simulink model "UnusedModels"  (R2015a)
settings: Solver=ode45  StartTime=0.0  StopTime=10.0  RelTol=1e-3
values from neighbouring files (symbols this model uses):
  car_params = Simulink_Car_params    [TV2016_parameters.m]
  energyLimitControl = Simulink_energyLimit    [TV2016_parameters.m]
  settings = Simulink_Settings    [TV2016_parameters.m]
  speedEstimation = Simulink_speedEst    [TV2016_parameters.m]
  tractionControl = Simulink_tc    [TV2016_parameters.m]
  yawRateControl = Simulink_yawRate    [TV2016_parameters.m]
undefined symbols (not defined in the file or in its folder): canChannel, Use_Estimated_velocity
libraries: canlib x44, CarMaker4SL x33, canmsglib x28, simulink x6
(part 2 of 4)

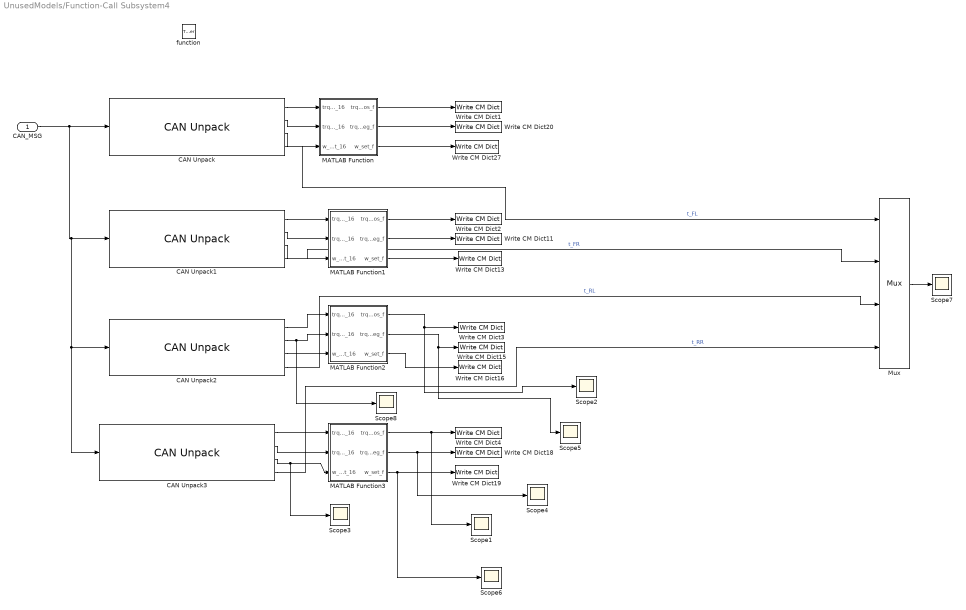
== system UnusedModels/Function-Call Subsystem4 ==
  CAN_MSG : Inport
  function : TriggerPort  TriggerType=function-call
  CAN Unpack : canmsglib/CAN Unpack  MsgList=(none)  MsgName=INV_FL  MsgIDType=Standard (11-bit identifier)  MsgIdentifier=CAN_ID_INV_FL  MsgLength=6  SignalInfo=trq_pos$0$16$1$1$1$0$1$0$-Inf$Inf$#trq_neg$16$16$1$1$1$0$1$0$-Inf$Inf$#w_set$32$16$1$1$1$0$1$0$-Inf$Inf$#  NSignals=3  IDPort=off  TimestampPort=on  ErrorPort=off  RemotePort=off  LengthPort=off  StatusPort=off  StartBits=str2num('[int32(0);int32(16);int32(32)]')  SignalSizes=str2num('[int32(16);int32(16);int32(16)]')  ByteOrders=str2num('[int32(1);int32(1);int32(1)]')  DataTypes=str2num('[int32(1);int32(1);int32(1)]')  MultiplexTypes=str2num('[int32(1);int32(1);int32(1)]')  MultiplexValues=str2num('[double(0);double(0);double(0)]')  Factors=str2num('[double(1);double(1);double(1)]')  Offsets=str2num('[double(0);double(0);double(0)]')  Minimums=str2num('[double(-Inf);double(-Inf);double(-Inf)]')  Maximums=str2num('[double(Inf);double(Inf);double(Inf)]')
  CAN Unpack1 : canmsglib/CAN Unpack  MsgList=(none)  MsgName=INV_FR  MsgIDType=Standard (11-bit identifier)  MsgIdentifier=CAN_ID_INV_FR  MsgLength=6  SignalInfo=trq_pos$0$16$1$1$1$0$1$0$-Inf$Inf$#trq_neg$16$16$1$1$1$0$1$0$-Inf$Inf$#w_set$32$16$1$1$1$0$1$0$-Inf$Inf$#  NSignals=3  IDPort=off  TimestampPort=on  ErrorPort=off  RemotePort=off  LengthPort=off  StatusPort=off  StartBits=str2num('[int32(0);int32(16);int32(32)]')  SignalSizes=str2num('[int32(16);int32(16);int32(16)]')  ByteOrders=str2num('[int32(1);int32(1);int32(1)]')  DataTypes=str2num('[int32(1);int32(1);int32(1)]')  MultiplexTypes=str2num('[int32(1);int32(1);int32(1)]')  MultiplexValues=str2num('[double(0);double(0);double(0)]')  Factors=str2num('[double(1);double(1);double(1)]')  Offsets=str2num('[double(0);double(0);double(0)]')  Minimums=str2num('[double(-Inf);double(-Inf);double(-Inf)]')  Maximums=str2num('[double(Inf);double(Inf);double(Inf)]')
  CAN Unpack2 : canmsglib/CAN Unpack  MsgList=(none)  MsgName=INV_RL  MsgIDType=Standard (11-bit identifier)  MsgIdentifier=CAN_ID_INV_RL  MsgLength=6  SignalInfo=trq_pos$0$16$1$1$1$0$1$0$-Inf$Inf$#trq_neg$16$16$1$1$1$0$1$0$-Inf$Inf$#w_set$32$16$1$1$1$0$1$0$-Inf$Inf$#  NSignals=3  IDPort=off  TimestampPort=on  ErrorPort=off  RemotePort=off  LengthPort=off  StatusPort=off  StartBits=str2num('[int32(0);int32(16);int32(32)]')  SignalSizes=str2num('[int32(16);int32(16);int32(16)]')  ByteOrders=str2num('[int32(1);int32(1);int32(1)]')  DataTypes=str2num('[int32(1);int32(1);int32(1)]')  MultiplexTypes=str2num('[int32(1);int32(1);int32(1)]')  MultiplexValues=str2num('[double(0);double(0);double(0)]')  Factors=str2num('[double(1);double(1);double(1)]')  Offsets=str2num('[double(0);double(0);double(0)]')  Minimums=str2num('[double(-Inf);double(-Inf);double(-Inf)]')  Maximums=str2num('[double(Inf);double(Inf);double(Inf)]')
  CAN Unpack3 : canmsglib/CAN Unpack  MsgList=(none)  MsgName=INV_RR  MsgIDType=Standard (11-bit identifier)  MsgIdentifier=CAN_ID_INV_RR  MsgLength=6  SignalInfo=trq_pos$0$16$1$1$1$0$1$0$-Inf$Inf$#trq_neg$16$16$1$1$1$0$1$0$-Inf$Inf$#w_set$32$16$1$1$1$0$1$0$-Inf$Inf$#  NSignals=3  IDPort=off  TimestampPort=on  ErrorPort=off  RemotePort=off  LengthPort=off  StatusPort=off  StartBits=str2num('[int32(0);int32(16);int32(32)]')  SignalSizes=str2num('[int32(16);int32(16);int32(16)]')  ByteOrders=str2num('[int32(1);int32(1);int32(1)]')  DataTypes=str2num('[int32(1);int32(1);int32(1)]')  MultiplexTypes=str2num('[int32(1);int32(1);int32(1)]')  MultiplexValues=str2num('[double(0);double(0);double(0)]')  Factors=str2num('[double(1);double(1);double(1)]')  Offsets=str2num('[double(0);double(0);double(0)]')  Minimums=str2num('[double(-Inf);double(-Inf);double(-Inf)]')  Maximums=str2num('[double(Inf);double(Inf);double(Inf)]')
  MATLAB Function : MATLAB Function  TreatAsAtomicUnit=on
  MATLAB Function1 : MATLAB Function  TreatAsAtomicUnit=on
  MATLAB Function2 : MATLAB Function  TreatAsAtomicUnit=on
  MATLAB Function3 : MATLAB Function  TreatAsAtomicUnit=on
  Mux : Mux
  Scope{1..8} (8 alike) : Scope
      Scope1 settings: YMin=0  YMax=11
      Scope2 settings: YMin=0  YMax=14
      Scope3 settings: YMin=-33196.8  YMax=30000  SaveName=ScopeData7
      Scope4 settings: YMin=0  YMax=11  SaveName=ScopeData2
      Scope5 settings: YMin=0  YMax=14  SaveName=ScopeData3
      Scope6 settings: YMin=0  YMax=11  SaveName=ScopeData6
      Scope7 settings: ShowLegends=on  TimeRange=9.572585353545549e-05  YMin=2742.34  YMax=2742.47  SaveName=ScopeData9
      Scope8 settings: YMin=0  YMax=14  SaveName=ScopeData13
  Write CM Dict1 : CarMaker4SL/Write CM Dict  xname=Tlim_pos_FL  xsync=off
  Write CM Dict11 : CarMaker4SL/Write CM Dict  xname=Tlim_neg_FR  xsync=off
  Write CM Dict13 : CarMaker4SL/Write CM Dict  xname=w_set_FR  xsync=off
  Write CM Dict15 : CarMaker4SL/Write CM Dict  xname=Tlim_neg_RL  xsync=off
  Write CM Dict16 : CarMaker4SL/Write CM Dict  xname=w_set_RL  xsync=off
  Write CM Dict18 : CarMaker4SL/Write CM Dict  xname=Tlim_neg_RR  xsync=off
  Write CM Dict19 : CarMaker4SL/Write CM Dict  xname=w_set_RR  xsync=off
  Write CM Dict2 : CarMaker4SL/Write CM Dict  xname=Tlim_pos_FR  xsync=off
  Write CM Dict20 : CarMaker4SL/Write CM Dict  xname=Tlim_neg_FL  xsync=off
  Write CM Dict27 : CarMaker4SL/Write CM Dict  xname=w_set_FL  xsync=off
  Write CM Dict3 : CarMaker4SL/Write CM Dict  xname=Tlim_pos_RL  xsync=off
  Write CM Dict4 : CarMaker4SL/Write CM Dict  xname=Tlim_pos_RR  xsync=off
  wires:
  CAN_MSG/1 -> CAN Unpack2/1, CAN Unpack3/1, CAN Unpack1/1, CAN Unpack/1
  CAN Unpack/2 -> MATLAB Function/2(trq_neg_16)
  CAN Unpack/3 -> MATLAB Function/3(w_set_16)
  CAN Unpack/1 -> MATLAB Function/1(trq_pos_16)
  MATLAB Function/1(trq_pos_f) -> Write CM Dict1/1
  MATLAB Function/2(trq_neg_f) -> Write CM Dict20/1
  MATLAB Function/3(w_set_f) -> Write CM Dict27/1
  CAN Unpack1/2 -> MATLAB Function1/2(trq_neg_16)
  CAN Unpack1/1 -> MATLAB Function1/1(trq_pos_16)
  CAN Unpack1/3 -> MATLAB Function1/3(w_set_16)
  MATLAB Function1/1(trq_pos_f) -> Write CM Dict2/1
  MATLAB Function1/2(trq_neg_f) -> Write CM Dict11/1
  MATLAB Function1/3(w_set_f) -> Write CM Dict13/1
  CAN Unpack2/1 -> MATLAB Function2/1(trq_pos_16)
  CAN Unpack2/2 -> Scope8/1, MATLAB Function2/2(trq_neg_16)
  CAN Unpack2/3 -> MATLAB Function2/3(w_set_16)
  MATLAB Function2/3(w_set_f) -> Write CM Dict16/1
  MATLAB Function2/2(trq_neg_f) -> Scope5/1, Write CM Dict15/1
  MATLAB Function2/1(trq_pos_f) -> Scope2/1, Write CM Dict3/1
  CAN Unpack3/1 -> MATLAB Function3/1(trq_pos_16)
  CAN Unpack3/2 -> MATLAB Function3/2(trq_neg_16)
  CAN Unpack3/3 -> Scope3/1, MATLAB Function3/3(w_set_16)
  MATLAB Function3/3(w_set_f) -> Scope6/1, Write CM Dict19/1
  MATLAB Function3/2(trq_neg_f) -> Scope4/1, Write CM Dict18/1
  MATLAB Function3/1(trq_pos_f) -> Scope1/1, Write CM Dict4/1
  CAN Unpack2/4 -> Mux/3  "t_RL"
  CAN Unpack/4 -> Mux/1  "t_FL"
  CAN Unpack1/4 -> Mux/2  "t_FR"
  CAN Unpack3/4 -> Mux/4  "t_RR"
  Mux/1 -> Scope7/1

== system UnusedModels/Fz_Estimation ==
  sensors : Inport
  FzCalc : Scope
      settings: ShowLegends=on  TimeRange=0.5129057337220599  YMin=982.0067255187187  YMax=982.99982331966  SaveName=ScopeData51
  FzEst : MATLAB Function  TreatAsAtomicUnit=on
  "deltaFz " : Scope
      settings: ShowLegends=on  TimeRange=10  YMin=-650  YMax=50  SaveName=ScopeData52
  lateral : Scope
      settings: ShowLegends=on  TimeRange=1.971383147853736  YMin=574.5308310991956  YMax=1245.308310991957  SaveName=ScopeData48
  vertialest : Scope
      settings: ShowLegends=on  TimeRange=10  YMin=-650  YMax=50  SaveName=ScopeData49
  Fz_est : Outport
  wires:
  sensors/1 -> FzEst/1(sensor)
  FzEst/2(x_out) -> lateral/1
  FzEst/3(xv_out) -> vertialest/1
  FzEst/4(FZ) -> FzCalc/1
  FzEst/5(delta_Fzl) -> "deltaFz "/1
  FzEst/1(normalForces) -> Fz_est/1

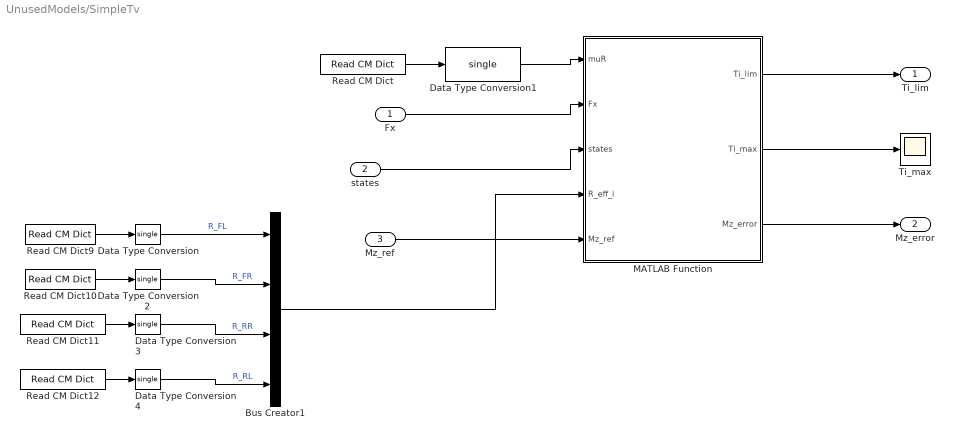
== system UnusedModels/SimpleTv ==
  Fx : Inport
  states : Inport  Port=2
  Mz_ref : Inport  Port=3
  Bus Creator1 : BusCreator  OutDataTypeStr=Bus: R_eff_i
  Data Type Conversion{,1..4} (5 alike) : DataTypeConversion  OutDataTypeStr=single
  MATLAB Function : MATLAB Function  TreatAsAtomicUnit=on
  Read CM Dict : CarMaker4SL/Read CM Dict  xname=Car.muRoadRL  xsync=off
  Read CM Dict10 : CarMaker4SL/Read CM Dict  xname=Car.WFR.Radius  xsync=off
  Read CM Dict11 : CarMaker4SL/Read CM Dict  xname=Car.WRR.Radius  xsync=off
  Read CM Dict12 : CarMaker4SL/Read CM Dict  xname=Car.WRL.Radius  xsync=off
  Read CM Dict9 : CarMaker4SL/Read CM Dict  xname=Car.WFL.Radius  xsync=off
  Ti_max : Scope
      settings: ShowLegends=on  TimeRange=1.803977272727272  YMin=0  YMax=17  SaveName=ScopeData25
  Ti_lim : Outport
  Mz_error : Outport  Port=2
  wires:
  Fx/1 -> MATLAB Function/2(Fx)
  states/1 -> MATLAB Function/3(states)
  Read CM Dict/1 -> Data Type Conversion1/1
  Data Type Conversion1/1 -> MATLAB Function/1(muR)
  MATLAB Function/1(Ti_lim) -> Ti_lim/1
  Read CM Dict9/1 -> Data Type Conversion/1
  Read CM Dict11/1 -> Data Type Conversion3/1
  Read CM Dict12/1 -> Data Type Conversion4/1
  Read CM Dict10/1 -> Data Type Conversion2/1
  Data Type Conversion4/1 -> Bus Creator1/4  "R_RL"
  Data Type Conversion2/1 -> Bus Creator1/2  "R_FR"
  Data Type Conversion3/1 -> Bus Creator1/3  "R_RR"
  Data Type Conversion/1 -> Bus Creator1/1  "R_FL"
  Bus Creator1/1 -> MATLAB Function/4(R_eff_i)
  Mz_ref/1 -> MATLAB Function/5(Mz_ref)
  MATLAB Function/2(Ti_max) -> Ti_max/1
  MATLAB Function/3(Mz_error) -> Mz_error/1

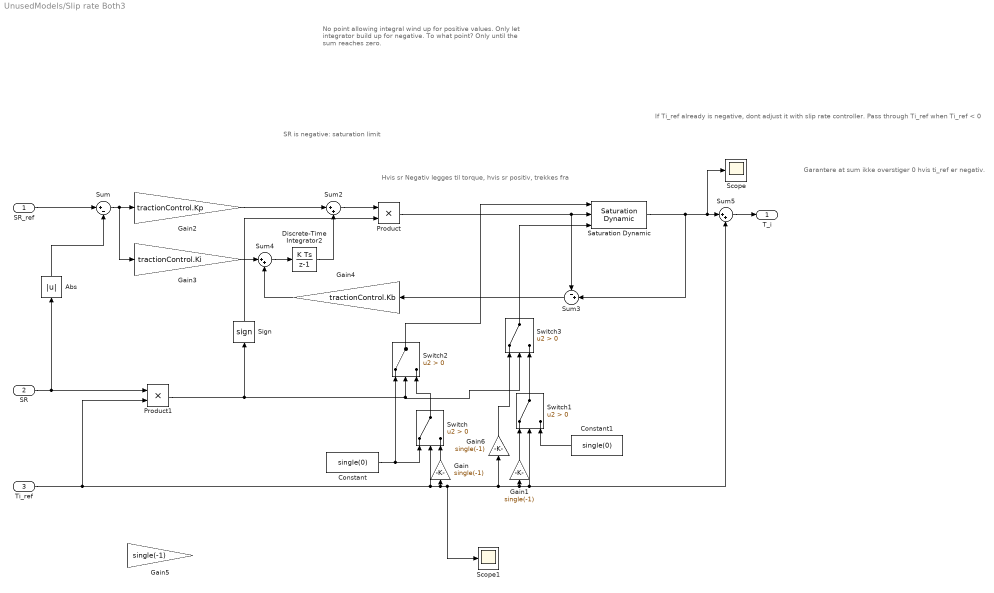
== system UnusedModels/Slip rate Both3 ==
  note: If Ti_ref already is negative, dont adjust it with slip rate controller. Pass through Ti_ref when Ti_ref < 0
  note: No point allowing integral wind up for positive values.
      | Only let integrator build up for negative. To what point?
      | Only until the sum reaches zero.
  note: Hvis sr Negativ legges til torque, hvis sr positiv, trekkes fra
  note: Garantere at sum ikke overstiger 0 hvis ti_ref er negativ.
  note: SR is negative: saturation limit
  SR_ref : Inport
  SR : Inport  Port=2
  Ti_ref : Inport  Port=3
  Abs : Abs
  Constant : Constant  Value=single(0)
  Constant1 : Constant  Value=single(0)
  Discrete-Time Integrator2 : DiscreteIntegrator  SampleTime=-1
  Gain{,1,5..6} (4 alike) : Gain  Gain=single(-1)
  Gain2 : Gain  Gain=tractionControl.Kp
  Gain3 : Gain  Gain=tractionControl.Ki
  Gain4 : Gain  Gain=tractionControl.Kb
  Product : Product
  Product1 : Product
  Saturation Dynamic : simulink/Discontinuities/Saturation Dynamic  OutMin=[]  OutMax=[]  OutDataTypeStr=Inherit: Same as second input  OutDataType=fixdt(1, 16)  OutScaling=2^-10  DoSatur=off
  Scope : Scope
      settings: ShowLegends=on  SaveName=ScopeData9
  Scope1 : Scope
      settings: ShowLegends=on  SaveName=ScopeData14
  Sign : Signum
  Sum : Sum  Inputs=|+-
  Sum2 : Sum  Inputs=|++
  Sum3 : Sum  Inputs=-+|
  Sum4 : Sum  Inputs=|++
  Sum5 : Sum  Inputs=|++
  Switch{,1..3} (4 alike) : Switch  Criteria=u2 > Threshold
  T_i : Outport
  wires:
  Abs/1 -> Sum/2
  Product/1 -> Sum3/1, Saturation Dynamic/2
  Sum2/1 -> Product/1
  Gain4/1 -> Sum4/2
  Sum4/1 -> Discrete-Time Integrator2/1
  Gain3/1 -> Sum4/1
  Sum3/1 -> Gain4/1
  Saturation Dynamic/1 -> Sum3/2, Scope/1, Sum5/1
  Discrete-Time Integrator2/1 -> Sum2/2
  Gain2/1 -> Sum2/1
  Sum/1 -> Gain2/1, Gain3/1
  Gain1/1 -> Switch1/1
  Constant1/1 -> Switch1/3
  Constant/1 -> Switch2/1, Switch/1
  Gain/1 -> Switch/3
  SR/1 -> Product1/1, Abs/1
  Sum5/1 -> T_i/1
  Ti_ref/1 -> Switch/2, Scope1/1, Gain1/1, Sum5/2, Switch1/2, Gain6/1, Gain/1, Product1/2
  SR_ref/1 -> Sum/1
  Product1/1 -> Switch3/2, Switch2/2, Sign/1
  Switch/1 -> Switch2/3
  Switch2/1 -> Saturation Dynamic/1
  Switch3/1 -> Saturation Dynamic/3
  Gain6/1 -> Switch3/1
  Switch1/1 -> Switch3/3
  ? -> ?
  ? -> ?
  Sign/1 -> Product/2

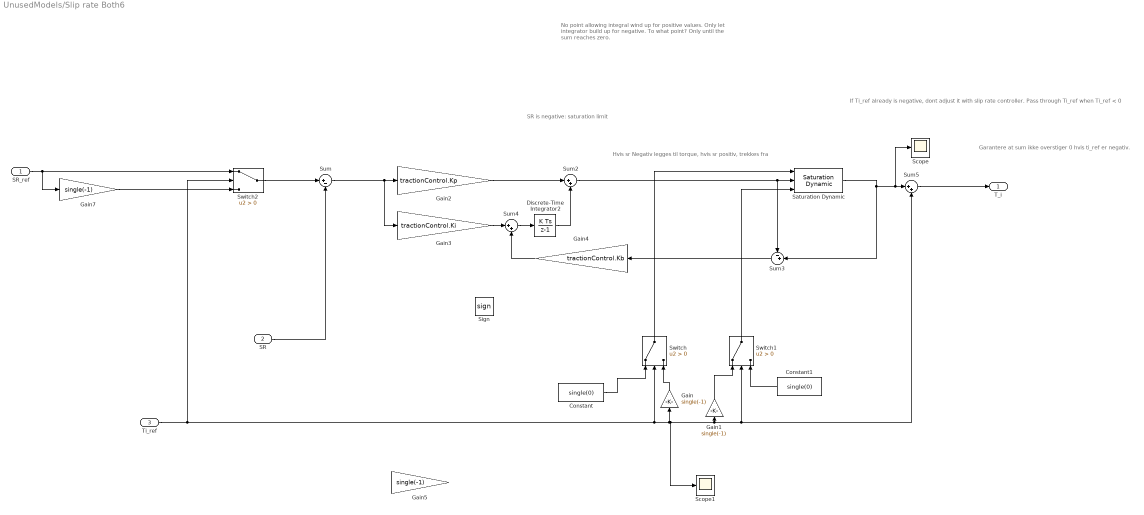
== system UnusedModels/Slip rate Both6 ==
  note: SR is negative: saturation limit
  note: Garantere at sum ikke overstiger 0 hvis ti_ref er negativ.
  note: Hvis sr Negativ legges til torque, hvis sr positiv, trekkes fra
  note: No point allowing integral wind up for positive values.
      | Only let integrator build up for negative. To what point?
      | Only until the sum reaches zero.
  note: If Ti_ref already is negative, dont adjust it with slip rate controller. Pass through Ti_ref when Ti_ref < 0
  SR_ref : Inport
  SR : Inport  Port=2
  Ti_ref : Inport  Port=3
  Constant : Constant  Value=single(0)
  Constant1 : Constant  Value=single(0)
  Discrete-Time Integrator2 : DiscreteIntegrator  SampleTime=-1
  Gain{,1,5,7} (4 alike) : Gain  Gain=single(-1)
  Gain2 : Gain  Gain=tractionControl.Kp
  Gain3 : Gain  Gain=tractionControl.Ki
  Gain4 : Gain  Gain=tractionControl.Kb
  Saturation Dynamic : simulink/Discontinuities/Saturation Dynamic  OutMin=[]  OutMax=[]  OutDataTypeStr=Inherit: Same as second input  OutDataType=fixdt(1, 16)  OutScaling=2^-10  DoSatur=off
  Scope : Scope
      settings: ShowLegends=on  SaveName=ScopeData9
  Scope1 : Scope
      settings: ShowLegends=on  SaveName=ScopeData14
  Sign : Signum
  Sum : Sum  Inputs=|+-
  Sum2 : Sum  Inputs=|++
  Sum3 : Sum  Inputs=-+|
  Sum4 : Sum  Inputs=|++
  Sum5 : Sum  Inputs=|++
  Switch : Switch  Criteria=u2 > Threshold
  Switch1 : Switch  Criteria=u2 > Threshold
  Switch2 : Switch  Criteria=u2 > Threshold
  T_i : Outport
  wires:
  Switch1/1 -> Saturation Dynamic/3
  Switch/1 -> Saturation Dynamic/1
  Switch2/1 -> Sum/1
  Gain7/1 -> Switch2/3
  SR_ref/1 -> Switch2/1, Gain7/1
  Ti_ref/1 -> Switch/2, Gain/1, Gain1/1, Switch1/2, Sum5/2, Scope1/1, Switch2/2
  Sum5/1 -> T_i/1
  Gain/1 -> Switch/3
  Constant/1 -> Switch/1
  Constant1/1 -> Switch1/3
  Gain1/1 -> Switch1/1
  Sum/1 -> Gain3/1, Gain2/1
  Gain2/1 -> Sum2/1
  Discrete-Time Integrator2/1 -> Sum2/2
  Saturation Dynamic/1 -> Sum5/1, Scope/1, Sum3/2
  Sum3/1 -> Gain4/1
  Gain3/1 -> Sum4/1
  Sum4/1 -> Discrete-Time Integrator2/1
  Gain4/1 -> Sum4/2
  Sum2/1 -> Saturation Dynamic/2, Sum3/1
  SR/1 -> Sum/2

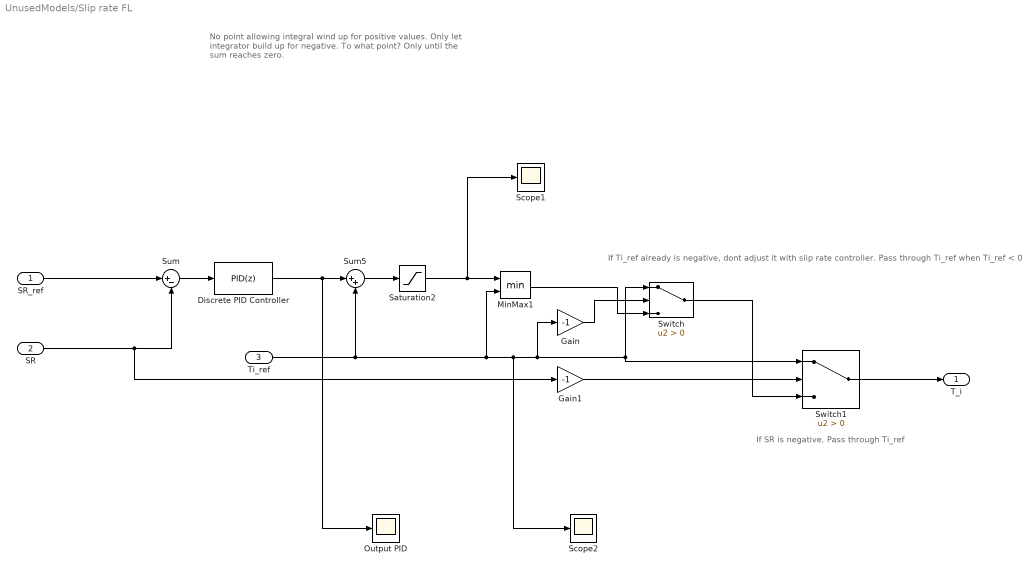
== system UnusedModels/Slip rate FL ==
  note: No point allowing integral wind up for positive values.
      | Only let integrator build up for negative. To what point?
      | Only until the sum reaches zero.
  note: If Ti_ref already is negative, dont adjust it with slip rate controller. Pass through Ti_ref when Ti_ref < 0
  note: If SR is negative. Pass through Ti_ref
  SR_ref : Inport
  SR : Inport  Port=2
  Ti_ref : Inport  Port=3
  Discrete PID Controller : simulink/Continuous/PID Controller  Controller=PID  TimeDomain=Discrete-time  SampleTime=-1  IntegratorMethod=Forward Euler  FilterMethod=Forward Euler  Form=Parallel  UseFilter=on  ControllerParametersSource=internal  P=tractionControl.Kp  I=tractionControl.Ki  D=tractionControl.Kd  N=100  InitialConditionSource=internal  InitialConditionForIntegrator=0  InitialConditionForFilter=0  ExternalReset=none  LimitOutput=on  UpperSaturationLimit=tractionControl.upper_sat_limit  LowerSaturationLimit=tractionControl.lower_sat_limit  LinearizeAsGain=off  AntiWindupMode=back-calculation  Kb=tractionControl.Kb  TrackingMode=off  Kt=1  PParamMin=[]  PParamMax=[]  IParamMin=[]  IParamMax=[]  DParamMin=[]  DParamMax=[]  NParamMin=[]  NParamMax=[]  KbParamMin=[]  KbParamMax=[]  KtParamMin=[]  KtParamMax=[]  POutMin=[]  POutMax=[]  IOutMin=[]  IOutMax=[]  DOutMin=[]  DOutMax=[]  NOutMin=[]  NOutMax=[]  KbOutMin=[]  KbOutMax=[]  KtOutMin=[]  KtOutMax=[]  IntegratorOutMin=[]  IntegratorOutMax=[]  FilterOutMin=[]  FilterOutMax=[]  SumOutMin=[]  SumOutMax=[]  SumI1OutMin=[]  SumI1OutMax=[]  SumI2OutMin=[]  SumI2OutMax=[]  SumI3OutMin=[]  SumI3OutMax=[]  SumDOutMin=[]  SumDOutMax=[]  SaturationOutMin=[]  SaturationOutMax=[]  IntegratorContinuousStateAttributes=''  IntegratorStateMustResolveToSignalObject=off  IntegratorRTWStateStorageClass=Auto  FilterContinuousStateAttributes=''  FilterStateMustResolveToSignalObject=off  FilterRTWStateStorageClass=Auto  DifferentiatorICPrevScaledInput=0  DifferentiatorOutMin=[]  DifferentiatorOutMax=[]
  Gain : Gain  Gain=-1
  Gain1 : Gain  Gain=-1
  MinMax1 : MinMax  Inputs=2
  Output PID : Scope
      settings: TimeRange=10  SaveName=ScopeData19
  Saturation2 : Saturate  UpperLimit=settings.max_motor_torque  LowerLimit=0
  Scope1 : Scope
      settings: TimeRange=10  SaveName=ScopeData9
  Scope2 : Scope
      settings: TimeRange=10  SaveName=ScopeData14
  Sum : Sum  Inputs=|+-
  Sum5 : Sum  Inputs=|++
  Switch : Switch  Criteria=u2 > Threshold
  Switch1 : Switch  Criteria=u2 > Threshold
  T_i : Outport
  wires:
  SR/1 -> Gain1/1, Sum/2
  SR_ref/1 -> Sum/1
  Sum/1 -> Discrete PID Controller/1
  Ti_ref/1 -> Switch/1, Switch1/1, Gain/1, Scope2/1, MinMax1/2, Sum5/2
  Sum5/1 -> Saturation2/1
  MinMax1/1 -> Switch/3
  Discrete PID Controller/1 -> Output PID/1, Sum5/1
  Gain/1 -> Switch/2
  Saturation2/1 -> Scope1/1, MinMax1/1
  Switch/1 -> Switch1/3
  Gain1/1 -> Switch1/2
  Switch1/1 -> T_i/1

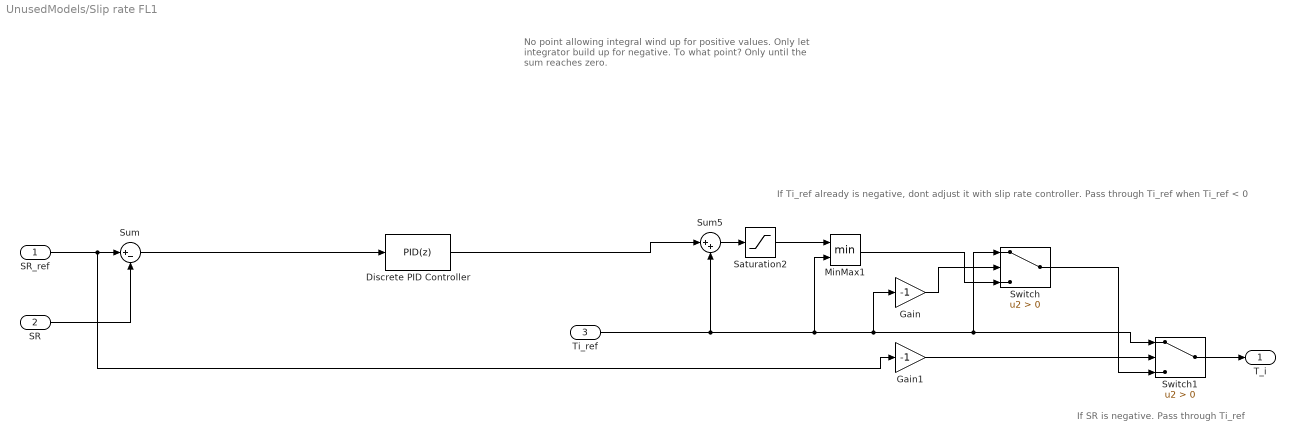
== system UnusedModels/Slip rate FL1 ==
  note: If SR is negative. Pass through Ti_ref
  note: If Ti_ref already is negative, dont adjust it with slip rate controller. Pass through Ti_ref when Ti_ref < 0
  note: No point allowing integral wind up for positive values.
      | Only let integrator build up for negative. To what point?
      | Only until the sum reaches zero.
  SR_ref : Inport
  SR : Inport  Port=2
  Ti_ref : Inport  Port=3
  Discrete PID Controller : simulink/Continuous/PID Controller  Controller=PID  TimeDomain=Discrete-time  SampleTime=-1  IntegratorMethod=Forward Euler  FilterMethod=Forward Euler  Form=Parallel  UseFilter=on  ControllerParametersSource=internal  P=tractionControl.Kp  I=tractionControl.Ki  D=tractionControl.Kd  N=100  InitialConditionSource=internal  InitialConditionForIntegrator=0  InitialConditionForFilter=0  ExternalReset=none  LimitOutput=on  UpperSaturationLimit=tractionControl.upper_sat_limit  LowerSaturationLimit=tractionControl.lower_sat_limit  LinearizeAsGain=off  AntiWindupMode=back-calculation  Kb=tractionControl.Kb  TrackingMode=off  Kt=1  PParamMin=[]  PParamMax=[]  IParamMin=[]  IParamMax=[]  DParamMin=[]  DParamMax=[]  NParamMin=[]  NParamMax=[]  KbParamMin=[]  KbParamMax=[]  KtParamMin=[]  KtParamMax=[]  POutMin=[]  POutMax=[]  IOutMin=[]  IOutMax=[]  DOutMin=[]  DOutMax=[]  NOutMin=[]  NOutMax=[]  KbOutMin=[]  KbOutMax=[]  KtOutMin=[]  KtOutMax=[]  IntegratorOutMin=[]  IntegratorOutMax=[]  FilterOutMin=[]  FilterOutMax=[]  SumOutMin=[]  SumOutMax=[]  SumI1OutMin=[]  SumI1OutMax=[]  SumI2OutMin=[]  SumI2OutMax=[]  SumI3OutMin=[]  SumI3OutMax=[]  SumDOutMin=[]  SumDOutMax=[]  SaturationOutMin=[]  SaturationOutMax=[]  IntegratorContinuousStateAttributes=''  IntegratorStateMustResolveToSignalObject=off  IntegratorRTWStateStorageClass=Auto  FilterContinuousStateAttributes=''  FilterStateMustResolveToSignalObject=off  FilterRTWStateStorageClass=Auto  DifferentiatorICPrevScaledInput=0  DifferentiatorOutMin=[]  DifferentiatorOutMax=[]
  Gain : Gain  Gain=-1
  Gain1 : Gain  Gain=-1
  MinMax1 : MinMax  Inputs=2
  Saturation2 : Saturate  UpperLimit=settings.max_motor_torque  LowerLimit=0
  Sum : Sum  Inputs=|+-
  Sum5 : Sum  Inputs=|++
  Switch : Switch  Criteria=u2 > Threshold
  Switch1 : Switch  Criteria=u2 > Threshold
  T_i : Outport
  wires:
  Switch1/1 -> T_i/1
  Gain1/1 -> Switch1/2
  Switch/1 -> Switch1/3
  Saturation2/1 -> MinMax1/1
  Gain/1 -> Switch/2
  MinMax1/1 -> Switch/3
  Sum5/1 -> Saturation2/1
  Ti_ref/1 -> Sum5/2, MinMax1/2, Gain/1, Switch1/1, Switch/1
  Sum/1 -> Discrete PID Controller/1
  SR_ref/1 -> Sum/1, Gain1/1
  SR/1 -> Sum/2
  Discrete PID Controller/1 -> Sum5/1

== system UnusedModels/speedEstimate ==
  sensors : Inport
  Fz_est_in : Inport  Port=2
  RPMDerivative : Inport  Port=3
  Mux : Mux  Inputs=6
  Vestimate : MATLAB Function  TreatAsAtomicUnit=on
  "Y_meas " : Scope
      settings: TimeRange=0.009610450985687358  YMin=14.58015804088158  YMax=14.75728217480567  SaveName=ScopeData41
  variances : Scope
      settings: ShowLegends=on  TimeRange=0.009014007770619354  YMin=0.003396802325581397  YMax=0.004260174418604652  SaveName=ScopeData45
  V_est_x : Outport
  whl_cog_speed : Outport  Port=2
  wires:
  Vestimate/1(V_est_x) -> V_est_x/1
  Vestimate/3(Y_meas) -> "Y_meas "/1
  Vestimate/4(front_rear_Var) -> Mux/1  "front_rear"
  Vestimate/5(front_Var) -> Mux/2  "front"
  Vestimate/6(rear_Var) -> Mux/3  "rear"
  Vestimate/7(all_Var) -> Mux/4  "total"
  Vestimate/8(left_Var) -> Mux/5  "left"
  Vestimate/9(right_Var) -> Mux/6  "right"
  Mux/1 -> variances/1
  sensors/1 -> Vestimate/1(sensors)
  RPMDerivative/1 -> Vestimate/2(RPM_derivative)
  Fz_est_in/1 -> Vestimate/3(normalForces)
  Vestimate/2(whl_speed) -> whl_cog_speed/1

== system UnusedModels/Estimations /Normal Force Direct Calculation ==
  Measurements : Inport
  MATLAB Function : MATLAB Function  TreatAsAtomicUnit=on
  Fz_FL : Outport
  Fz_FR : Outport  Port=2
  Fz_RL : Outport  Port=3
  Fz_RR : Outport  Port=4
  wires:
  Measurements/1 -> MATLAB Function/1(sensor)
  MATLAB Function/1(Fz_FL) -> Fz_FL/1
  MATLAB Function/2(Fz_FR) -> Fz_FR/1
  MATLAB Function/3(Fz_RL) -> Fz_RL/1
  MATLAB Function/4(Fz_RR) -> Fz_RR/1

== system UnusedModels/Estimations /Normal Force Kalman Filters ==
  Measurements : Inport
  FzCalc : Scope
      settings: ShowLegends=on  TimeRange=0.5129057337220599  YMin=982.0067255187187  YMax=982.99982331966  SaveName=ScopeData51
  MATLAB Function : MATLAB Function  TreatAsAtomicUnit=on
  "deltaFz " : Scope
      settings: ShowLegends=on  TimeRange=10  YMin=-650  YMax=50  SaveName=ScopeData52
  lateral : Scope
      settings: ShowLegends=on  TimeRange=1.971383147853736  YMin=574.5308310991956  YMax=1245.308310991957  SaveName=ScopeData48
  vertialest : Scope
      settings: ShowLegends=on  TimeRange=10  YMin=-650  YMax=50  SaveName=ScopeData49
  Fz_FL : Outport
  Fz_FR : Outport  Port=2
  Fz_RL : Outport  Port=3
  Fz_RR : Outport  Port=4
  wires:
  Measurements/1 -> MATLAB Function/1(sensor)
  MATLAB Function/5(x_out) -> lateral/1
  MATLAB Function/6(xv_out) -> vertialest/1
  MATLAB Function/7(FZ) -> FzCalc/1
  MATLAB Function/8(delta_Fzl) -> "deltaFz "/1
  MATLAB Function/4(Fz_RR) -> Fz_RR/1
  MATLAB Function/3(Fz_RL) -> Fz_RL/1
  MATLAB Function/2(Fz_FR) -> Fz_FR/1
  MATLAB Function/1(Fz_FL) -> Fz_FL/1

== system UnusedModels/Estimations /RPM to wheel x velocities ==
  Measurements : Inport
  Calculate velocity of each wheel : MATLAB Function  TreatAsAtomicUnit=on
  FL : Outport
  FR : Outport  Port=2
  RL : Outport  Port=3
  RR : Outport  Port=4
  wires:
  Measurements/1 -> Calculate velocity of each wheel/1(sensor)
  Calculate velocity of each wheel/1(Whl_v_FL) -> FL/1
  Calculate velocity of each wheel/2(Whl_v_FR) -> FR/1
  Calculate velocity of each wheel/3(Whl_v_RL) -> RL/1
  Calculate velocity of each wheel/4(Whl_v_RR) -> RR/1

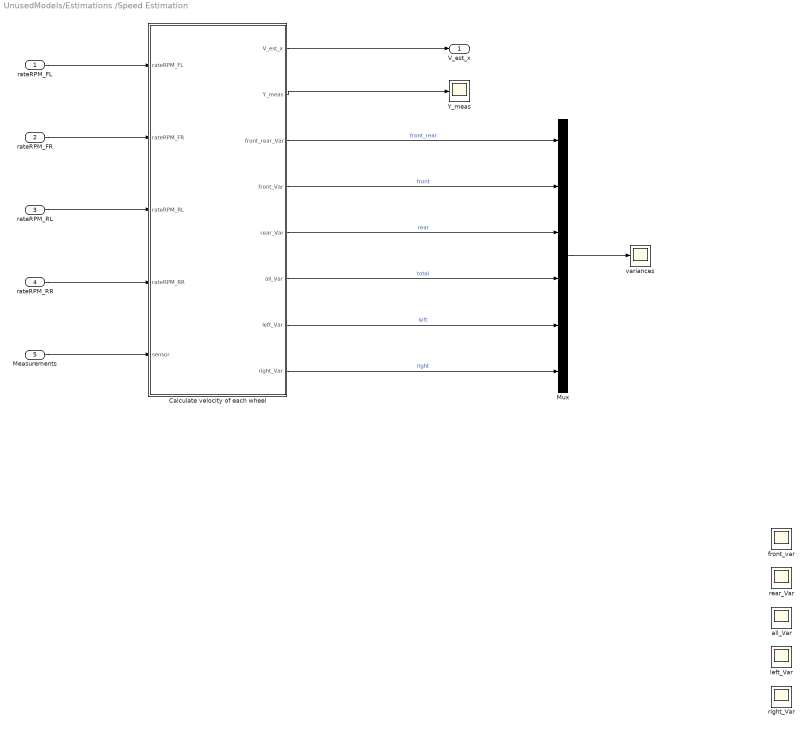
== system UnusedModels/Estimations /Speed Estimation ==
  rateRPM_FL : Inport
  rateRPM_FR : Inport  Port=2
  rateRPM_RL : Inport  Port=3
  rateRPM_RR : Inport  Port=4
  Measurements : Inport  Port=5
  Calculate velocity of each wheel : MATLAB Function  TreatAsAtomicUnit=on
  Mux : Mux  Inputs=6
  "Y_meas " : Scope
      settings: TimeRange=0.009610450985687358  YMin=14.58015804088158  YMax=14.75728217480567  SaveName=ScopeData41
  all_Var : Scope
      settings: TimeRange=0.5212732919254659  YMin=5e-05  YMax=0.00035  SaveName=ScopeData44
  front_var : Scope
      settings: TimeRange=0.5212732919254659  YMin=1.05879e-22  YMax=2.5e-06  SaveName=ScopeData53
  left_Var : Scope
      settings: TimeRange=0.5212732919254659  YMin=5e-05  YMax=0.00035  SaveName=ScopeData61
  rear_Var : Scope
      settings: TimeRange=10  YMin=5e-05  YMax=0.00035  SaveName=ScopeData54
  right_Var : Scope
      settings: TimeRange=0.5212732919254659  YMin=5e-05  YMax=0.00035  SaveName=ScopeData63
  variances : Scope
      settings: ShowLegends=on  TimeRange=0.009014007770619354  YMin=0.003396802325581397  YMax=0.004260174418604652  SaveName=ScopeData45
  V_est_x : Outport
  wires:
  Measurements/1 -> Calculate velocity of each wheel/5(sensor)
  Calculate velocity of each wheel/1(V_est_x) -> V_est_x/1
  Calculate velocity of each wheel/2(Y_meas) -> "Y_meas "/1
  Calculate velocity of each wheel/3(front_rear_Var) -> Mux/1  "front_rear"
  Calculate velocity of each wheel/4(front_Var) -> Mux/2  "front"
  Calculate velocity of each wheel/5(rear_Var) -> Mux/3  "rear"
  Calculate velocity of each wheel/6(all_Var) -> Mux/4  "total"
  Calculate velocity of each wheel/7(left_Var) -> Mux/5  "left"
  Calculate velocity of each wheel/8(right_Var) -> Mux/6  "right"
  Mux/1 -> variances/1
  rateRPM_FL/1 -> Calculate velocity of each wheel/1(rateRPM_FL)
  rateRPM_FR/1 -> Calculate velocity of each wheel/2(rateRPM_FR)
  rateRPM_RL/1 -> Calculate velocity of each wheel/3(rateRPM_RL)
  rateRPM_RR/1 -> Calculate velocity of each wheel/4(rateRPM_RR)

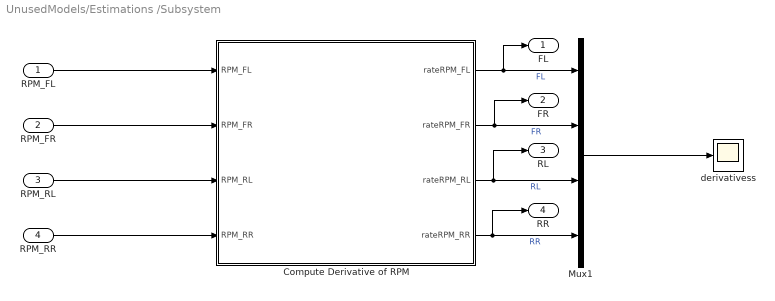
== system UnusedModels/Estimations /Subsystem ==
  RPM_FL : Inport
  RPM_FR : Inport  Port=2
  RPM_RL : Inport  Port=3
  RPM_RR : Inport  Port=4
  Compute Derivative of RPM : MATLAB Function  TreatAsAtomicUnit=on
  Mux1 : Mux
  "derivativess " : Scope
      settings: TimeRange=0.1259141104294481  YMin=5836.092715231789  YMax=6250  SaveName=ScopeData71
  FL : Outport
  FR : Outport  Port=2
  RL : Outport  Port=3
  RR : Outport  Port=4
  wires:
  RPM_FL/1 -> Compute Derivative of RPM/1(RPM_FL)
  RPM_FR/1 -> Compute Derivative of RPM/2(RPM_FR)
  RPM_RL/1 -> Compute Derivative of RPM/3(RPM_RL)
  RPM_RR/1 -> Compute Derivative of RPM/4(RPM_RR)
  Compute Derivative of RPM/3(rateRPM_RL) -> RL/1, Mux1/3  "RL"
  Compute Derivative of RPM/1(rateRPM_FL) -> FL/1, Mux1/1  "FL"
  Compute Derivative of RPM/2(rateRPM_FR) -> FR/1, Mux1/2  "FR"
  Compute Derivative of RPM/4(rateRPM_RR) -> RR/1, Mux1/4  "RR"
  Mux1/1 -> "derivativess "/1

== matlab function UnusedModels/Estimations /Normal Force Kalman Filters/MATLAB Function ==
  data: Fz_FL output; Fz_FR output; Fz_RL output; Fz_RR output; sensor input; settings parameter; car_params parameter; x_out output; xv_out output; FZ output; delta_Fzl output
function [Fz_FL, Fz_FR, Fz_RL ,Fz_RR, x_out,xv_out,FZ,delta_Fzl] = normalForceEstimation(sensor, settings,car_params)
%#codegen

te = settings.control_system_sample_time;

ms = car_params.sprung_mass; 
mv = car_params.mass; % Total mass( driver + car)
l = car_params.l; %Wheel base
lr = car_params.l_r;
lf = car_params.l_f;
hr = car_params.h_r;
hf = car_params.h_f;
ef = car_params.t_f*2; % Front track
er = car_params.t_r*2; % Rear track
kf = car_params.roll_stiff_f;
kr = car_params.roll_stiff_r;
Ixx = car_params.Ixx;
hcr = car_params.h_cr;
Kr = car_params.K_r;
Cr = car_params.C_r;
hc = car_params.CoG_height;
g = 9.81;


%ODFzL = linear lateral
%OFzE = nonlinear vertical
%OFzL = linear vertical


%State vector
A = zeros(5,5);
H = zeros(5,5);
A = single([1 0 -2*te*(ms/l)*( (lr*hf)/ef + (lf*hr)/er) 0 -2*te*(kf/ef + kr/er);
     0 1 te 0 0;
     0 0 1 0 0;
     0 0 0 1 te;
     0 te*ms*hcr/Ixx 0 te*(ms*g*hcr - Kr)/Ixx  (1+te*(-Cr)/Ixx)]);
%Only use roll rate measurement
%A = single([1 0 -2*te*(ms/l)*( (lr*hf)/ef + (lf*hr)/er) 0 -2*te*(kf/ef + kr/er);
%    0 1 te 0 0;
%    0 0 1 0 0;
%    0 0 0 1 te;
%    0 0 0 0 0]);

% PS: If we measure true linear compensated ay, we dont need to
% adjust with roll angle or gravity. Just double check this.
H = single([0 1 0 0 0;
    0 0 0 1 0;
    0 0 0 0 1;
    1 0 0 0 0]);
%-------------------------------------------------------%
%-------------------------Lateral LKF-------------------%
%-------------------------------------------------------%
persistent firstIteration;
persistent x;
persistent P;

%State Vector: x = [left load transfer , ay_k , der_ay_k , rollAngle, rollRate]
%Measurement vector = [aym, rollAngle, rollRate, left load transfer meas]

%Q = single(diag([1000, 0.1, 0.1, 0.1, 0.1])); % Book parameters
% Notice that last state is weighted very low since there is no process
Q = single(diag([1000, 0.1, 0.1, 0.1, 0.001])); % Book parameters

R = single( diag([0.01 0.01 0.01 100])); % Taken from book

K = single(zeros(5,4));

x_out = single(zeros(5,1));
delta_Fzl = single(0);
if isempty(firstIteration)
    %firstIteration = 2; % Avoid overflow in the register and count 1 again
    %First time the function is called
    %Initialize
    P = single(eye(5));
    x = single(zeros(5,1)); % Also initial value
    x_out = x;
else
	x = A*x; % Prediction of the state
    P = A*P*A' + Q; % Predicted covariance
    
    %Measurement Update
    K = P*H'*inv(H*P*H' + R); % The filter gain
    Y_predicted = H*x; % Predicted measurement
    
    delta_Fzl = -2*(kf/ef + kr/er)*sensor.roll_angle - 2*ms*(sensor.ay/l)*(lr*hf/ef + lf*hr/er);
    Y_meas      = [sensor.ay; sensor.roll_angle; sensor.roll_rate; delta_Fzl];
    
    e = Y_meas - Y_predicted; %Difference between the measurement and predicted measurement 
    x = x + K*e; % Corrected state estimate
    x_out = x;
    P = P - K*H*P;
end

%-------------------------------------------------------%
%-------------------------Vertical Force LKF------------%
%-------------------------------------------------------%
%Assumes superposition principle. Change from LKF to EKF when time
a = te*(-mv*hc)/(2*l);
b = te*(-lr*mv*hc)/(l*ef);
br = te*(-lf*mv*hc)/(l*er);
Av = single([1 0 0 0 0 a 0 b;
            0 1 0 0 0 a 0 -b;
            0 0 1 0 0 -a 0 br;
            0 0 0 1 0 -a 0 -br;
            0 0 0 0 1 te 0 0;
            0 0 0 0 0 1 0 0;
            0 0 0 0 0 0 1 te;
            0 0 0 0 0 0 0 1]);
Hv = single([1 -1 1 -1 0 0 0 0;
            1 1 0 0 0 0 0 0;
            0 0 0 0 1 0 0 0;
            0 0 0 0 0 0 1 0;
            1 1 1 1 0 0 0 0]);
persistent xv;
persistent Pv;


Qv = single(diag([100 100 100 100 0.1 0.001 0.1 0.001])); % From book
Rv = single(diag([0.1 100 0.01 0.01 100])); % Taken from book( VehicleDynest)
Kv = single(zeros(8,5));      % Kalman gain

xv_out = single(zeros(8,1));
Y_measv = single(zeros(5,1));
Y_predictedv = single(zeros(5,1));

%-----------------------------------
%Normal force each tire calculcation
%-----------------------------------
%-----------------------------------
%Normal force each tire calculcation 2
%-----------------------------------
Fz11 = 0.5*mv*(lr*g/l - hc*sensor.ax/l) - mv*(lr*g/l - hc*sensor.ax/l)*hc*sensor.ay/(ef*g);
Fz12 = 0.5*mv*(lr*g/l - hc*sensor.ax/l) + mv*(lr*g/l - hc*sensor.ax/l)*hc*sensor.ay/(ef*g);

Fz21 = 0.5*mv*(lf*g/l + hc*sensor.ax/l) - mv*(lf*g/l + hc*sensor.ax/l)*hc*sensor.ay/(er*g);
Fz22 = 0.5*mv*(lf*g/l + hc*sensor.ax/l) + mv*(lf*g/l + hc*sensor.ax/l)*hc*sensor.ay/(er*g);

FZ = [Fz11; Fz12; Fz21; Fz22];

% Output:
Fz_FL = single(0);
Fz_FR = single(0);
Fz_RL = single(0);
Fz_RR = single(0);



% qf1 = 0.5*mv*(lr*g/l - hc*sensor.a_x/l);
% qf2 = mv*(lr*g/l - hc*sensor.a_x/l)*hc*sensor.a_y/(ef*g);
% Fz11 = qf1 - qf2; % sensor a_y or estimated a_y ????
% Fz12 = qf1 + qf2;
%FzObs = single(mv*(lr*g/l - hc*sensor.ax/l));
FzObs = single( Fz11 + Fz12);
mxx = single(mv*g/4);
sum_Fz = single(mv*g);
if isempty(firstIteration)
    firstIteration = 2; % Avoid overflow in the register and count 1 again
    %First time the function is called
    %Initialize
    xv = [mxx; mxx; mxx; mxx; 0; 0; 0; 0];
    Pv = single(eye(8));
    xv_out = xv;
else
	xv = Av*xv; % Prediction of the state
    Pv = Av*Pv*Av' + Qv; % Predicted covariance
    
    %Measurement Update
    Kv = Pv*Hv'/(Hv*Pv*Hv' + Rv); % The filter gain
    Y_predictedv = Hv*xv; % Predicted measurement
    
    Y_measv      = [x(1); FzObs; sensor.ax; x(2); sum_Fz];
    %x(1) = delta_Fzl from other observer
    %x(2) = estimated lateral acceleration compensating for roll angle
    ev = Y_measv - Y_predictedv; %Difference between the measurement and predicted measurement 
    xv = xv + Kv*ev; % Corrected state estimate
    xv_out = xv;
    Pv = Pv - Kv*Hv*Pv;
    Fz_FL = xv_out(1);
    Fz_FR = xv_out(2);
    Fz_RL = xv_out(3);
    Fz_RR = xv_out(4);
    
    
end

== matlab function UnusedModels/Estimations /Speed Estimation/Calculate velocity of each wheel ==
  data: rateRPM_FL input; rateRPM_FR input; rateRPM_RL input; rateRPM_RR input; sensor input; V_est_x output; settings parameter; car_params parameter; Y_meas output; front_rear_Var output; front_Var output; rear_Var output; all_Var output; left_Var output; right_Var output
function [V_est_x, Y_meas,front_rear_Var,front_Var,rear_Var,all_Var,left_Var,right_Var]...
         = SpeedEstimation(rateRPM_FL, rateRPM_FR,rateRPM_RL,rateRPM_RR,sensor,settings,car_params)
%#codegen

% ------------------------------
% DECLARATIONS
% ------------------------------
persistent firstIteration;
persistent v;
persistent error;
persistent K;
k_FL = single(0); % Gain 
k_FR = single(0); % Gain
k_RL = single(0); % Gain
k_RR = single(0); % Gain
% Gains for trusting, not trusting wheel speed measurements
Hg = settings.High_gain;
Lg = settings.Low_gain;
% Variances
all_Var = single(0); % Variance for all measurements
front_rear_Var = single(0);
front_Var = single(0);
rear_Var = single(0);
left_Var = single(0);
right_Var = single(0);
% LIMITS:
velocity_deviation_limit = settings.velocity_deviation_limit;
lim = settings.variance_limit;
RPM_derivative_limit = settings.RPM_derivative_limit;

% Measurement vector
C = [1;1;1;1]; % Create four copies of predicted vx


% ------------------------------
% PARAMETERS
% ------------------------------
%Conversion from RPM to rad/s for the wheel
c = single(2*pi/(car_params.GR*60));
t = settings.control_system_sample_time;
%Weights taken from wikipedia
%sg_Weight = single( [ 1; -8; 0; 8; -1] );
sg_Weight = single( [ -1; 8; 0; -8; 1] );
%sg_Weight = single([0.3; 0.1; -0.1 ; -0.3]);
%sg_Weight = single([1; -1; 0 ; -0]);
% ------------------------------
% COPY VARIABLES EACH TIMESTEP
% ------------------------------
S = sensor.Input_steering; % Steering angle in rad( Mean of front wheels)
ax = sensor.ax; % Should be true linear acceleration compensated for roll angle
%Fz, used to determine what wheel speeds to trust.
Fz = [sensor.Input_Fz_FL, sensor.Input_Fz_FR, sensor.Input_Fz_RL, sensor.Input_Fz_RR];
% Determine CoG Vx from motor RPM. Simple atm. Not considering vy.
Whl_v_FL = sensor.RPM_FL*c*car_params.r_eff*cos(S) + sensor.r*car_params.t_f;
Whl_v_FR = sensor.RPM_FR*c*car_params.r_eff*cos(S) - sensor.r*car_params.t_f;
Whl_v_RL = sensor.RPM_RL*c*car_params.r_eff + sensor.r*car_params.t_r;
Whl_v_RR = sensor.RPM_RR*c*car_params.r_eff - sensor.r*car_params.t_r;
RPM = [sensor.RPM_FL, sensor.RPM_FR, sensor.RPM_RL, sensor.RPM_RR]';
% Measurement vector, compensated RPMS
Y_meas = [Whl_v_FL, Whl_v_FR, Whl_v_RL, Whl_v_RR]';
% Different sums of normal forces, used to determine what wheels to trust
left_Fz = sum(Fz([1 3]));
right_Fz = sum(Fz([2 4]));
front_Fz = sum(Fz(1:2));
rear_Fz = sum(Fz(3:4));

% ------------------------------
% ESTIMATE DERIVATIVE OF COMPENSATED MOTOR RPM
% ------------------------------
% Problem with noise from yaw rate coupling into the derivative.. 
% Can I use uncompensated front wheels ? Should not be slipping like crazy
% with a significant steering angle ? 

% First try is with pure RPMS
% rateRPM_FL = simpleNumericalDerivative_RPM(sensor.RPM_FL,t);
% rateRPM_FR = simpleNumericalDerivative_RPM(sensor.RPM_FR,t);
% rateRPM_RL = simpleNumericalDerivative_RPM(sensor.RPM_RL,t);
% rateRPM_RR = simpleNumericalDerivative_RPM(sensor.RPM_RR,t);


% ------------------------------
% DRIFTING INS VELOCITY
% ------------------------------
persistent drift;




% ALGORITHM
if isempty(firstIteration)
    K = single(ones(1,4));
    v = single(0);
    V_est_x = v;
    error = Y_meas- C*v;
    firstIteration = 2;
    drift = single(0);
else
    drift = drift + 0.03*t;
    v_ins = sensor.V_x + 0.05 + drift;
    v = v + t*ax;
    %v = v + t*(ax + K*error);
    error = Y_meas - C*v ;
    V_est_x = 0.98*v;
    
    % Find K
    % Divide by zero problems...
    mean_WhlV = max(0.001,mean(Y_meas));
    mean_front_WhlV = max(0.001,mean(Y_meas(1:2)));
    mean_rear_WhlV  = max(0.001,mean(Y_meas(3:4)));
    mean_left_WhlV  = max(0.001,mean(Y_meas([1 3])));
    mean_right_WhlV = max(0.001,mean(Y_meas([2 4])));

    all_Var = var(Y_meas,1)/mean_WhlV;
    front_rear_Var = var([mean_front_WhlV, mean_rear_WhlV],1)/mean_WhlV;
    front_Var = var(Y_meas(1:2),1)/mean_front_WhlV;
    rear_Var  = var(Y_meas(3:4),1)/mean_rear_WhlV;
    
    left_Var    = var(Y_meas([1 3]),1)/mean_left_WhlV;
    right_Var   = var(Y_meas([2 4]),1)/mean_right_WhlV;   
    
    if (  (abs(Whl_v_FL - v_ins) > velocity_deviation_limit)...
       && (abs(Whl_v_FR - v_ins) > velocity_deviation_limit)...
       && (abs(Whl_v_RL - v_ins) > velocity_deviation_limit)...
       && (abs(Whl_v_RR - v_ins) > velocity_deviation_limit) )
        
        K = [Lg, Lg, Lg, Lg];
    
    elseif (all_Var  < lim ) 
        % low variance for all wheels.
        % Check derivative of motor RPM
        if ( (rateRPM_FL > RPM_derivative_limit) ||...
             (rateRPM_FR > RPM_derivative_limit) ||...
             (rateRPM_RL > RPM_derivative_limit) ||...
             (rateRPM_RR > RPM_derivative_limit))
            K = [Lg, Lg, Lg, Lg];
        % Rate of change of RPM can be low but slip rate is large
        % Check against drifting INS velocity 
        else
            K = [Hg, Hg ,Hg ,Hg];
        end
    % Variance is high. What wheel(s) are causing this.. 
    % STRUCTURE:
    % 1 = FRONT AND REAR DIFFER
    % 2 = LEFT AND RIGHT DIFFER
    % 3 = FL WRONG
    % 4 = FR WRONG
    % 5 = RL WRONG
    % 6 = RR WRONG
    % 7 Combinations of 3-6 that are not handled in 1-2.
    
    %1: FRONT AND REAR DIFFER
    elseif( (right_Var > front_Var) && (right_Var > rear_Var)...
            && (left_Var > front_Var) && (left_Var > rear_Var))
        % High variance between front and rear, and low variance 
        % at front and rear.
        
        % Also need to check if front/rear wheels are slipping
        
        % Front wheels over limit while rear is ok
        if (((rateRPM_FL > RPM_derivative_limit) ||...
             (rateRPM_FR > RPM_derivative_limit)) &&...
            ((rateRPM_RL < RPM_derivative_limit) ||...
             (rateRPM_RR < RPM_derivative_limit)) )
             
            K = [Lg, Lg, Hg, Hg];
        % Rear wheels over limit while front is ok
        elseif ( ((rateRPM_FL < RPM_derivative_limit) ||...
                 (rateRPM_FR < RPM_derivative_limit)) &&...
                ((rateRPM_RL > RPM_derivative_limit) ||...
                 (rateRPM_RR > RPM_derivative_limit)) )
             K = [Hg, Hg, Lg, Lg];
        % All are over limit
        elseif  ((rateRPM_FL > RPM_derivative_limit) &&...
                 (rateRPM_FR > RPM_derivative_limit) &&...
                 (rateRPM_RL > RPM_derivative_limit) &&...
                 (rateRPM_RR > RPM_derivative_limit) ) 
              K = [Lg, Lg, Lg, Lg];
              
        % The rate of change of RPM will flatten out and the high
        % slip ratio will still exist. Handle this
        
        % Check big difference in wheel speeds
        % Two cases. Driving and braking. 
        
        % Driving. Need logic to determine driving/braking
        elseif ( (RPM(1) + RPM(2)) > (RPM(3) + RPM(4)) )
            K = [Lg, Lg, Hg, Hg];
        elseif ( (RPM(1) + RPM(2)) < (RPM(3) + RPM(4)) )
            K = [Hg, Hg, Lg, Lg];
            % If frontFZ - rearFZ < 0, then FL is set to 0
            % Else it is set to a positive gain
%             k_FL = (1/abs(front_Fz-rear_Fz))*max(0,front_Fz - rear_Fz);
%             k_FR = (1/abs(front_Fz-rear_Fz))*max(0,front_Fz - rear_Fz);
% 
%             k_RL = (1/abs(rear_Fz-front_Fz))*max(0,rear_Fz-front_Fz)*0.5;
%             k_RR = (1/abs(rear_Fz-front_Fz))*max(0,rear_Fz-front_Fz)*0.5;
%            K = [k_FL, k_FR, k_RL, k_RR];
        end
    %2: LEFT AND RIGHT WHEELS DIFFER
    elseif ( ((front_Var > right_Var) && (rear_Var > right_Var)) ||...
            ( (front_Var > left_Var) && (rear_Var > left_Var)))
   
        k_FL = (1/abs(left_Fz-right_Fz))*max(0,left_Fz - right_Fz);
        k_RL = (1/abs(left_Fz-right_Fz))*max(0,left_Fz - right_Fz);
        
        k_FR = (1/abs(right_Fz-left_Fz))*max(0,right_Fz-left_Fz);
        k_RR = (1/abs(right_Fz-left_Fz))*max(0,right_Fz-left_Fz);
        
        K = [k_FL, k_FR, k_RL, k_RR];
        
    %3: FL WRONG
    elseif ( (left_Var > rear_Var) && (left_Var > right_Var)...
            && (front_Var > rear_Var) )
        k_FL = single(0);
        k_FR = single(0);
        k_RL = single(1);
        k_RR = single(1);
        K = [k_FL, k_FR, k_RL, k_RR];
    %4: FR WRONG
    elseif ( (right_Var > rear_Var) && (right_Var > left_Var)...
            && (front_Var > rear_Var))
        k_FL = single(0);
        k_FR = single(0);
        k_RL = single(1);
        k_RR = single(1);
        K = [k_FL, k_FR, k_RL, k_RR]; 
    %5: RL WRONG
    elseif ( (left_Var > front_Var) && (left_Var > right_Var)...
            && (rear_Var > front_Var))
        
        k_FL = single(1);
        k_FR = single(1);
        k_RL = single(0);
        k_RR = single(0);
        K = [k_FL, k_FR, k_RL, k_RR]; 
        
    %5: RR WRONG    
    elseif ( (right_Var > front_Var) && (right_Var > left_Var)...
            && (rear_Var > front_Var))
        k_FL = single(1);
        k_FR = single(1);
        k_RL = single(0);
        k_RR = single(0);
        K = [k_FL, k_FR, k_RL, k_RR]; 
    else
        k_FL = single(0);
        k_FR = single(0);
        k_RL = single(0);
        k_RR = single(0);
        K = [k_FL, k_FR, k_RL, k_RR]; 
    end
   
end
end

% function rateRPM = simpleNumericalDerivative_RPM(RPM, ts)
%     persistent firstIteration;
%     persistent RPM_prev;
%     
%     if isempty(firstIteration)
%         firstIteration = 2;
%         RPM_prev = RPM;
%         rateRPM = single(0);
%     else
%         %Calculate output
%         rateRPM = abs( (RPM - RPM_prev)/(ts));
%         RPM_prev = RPM;
%         if (rateRPM > 1000000)
%             rateRPM = single(0);
%         end
%     end    
% end



% function rateRPM = savitzkyGolay_RPM(RPM,nr_Coefficients,weight_Vector,ts)
%     % y(k) is rate of change of input variable per time step (ts) 
%     % means divide y(k) by ts 
%     % RPM is 4x1
%     % Weight vector is 4x1
%     persistent firstIteration;
%     persistent frame;
%  
%     % Filter at midpoint of dataset
%     % Assume even filter coeffs
%     midPoint = uint32(nr_Coefficients);
%     
%     % Declare
%     
%     rateRPM = single(0);
% 
%     if isempty(firstIteration)
%         firstIteration = 2;
%         frame = single(zeros(1,nr_Coefficients));
%         rateRPM = single(0);
%     else
%         %Update frame
%         % Newest first, discard last element
%         frame = [RPM, frame(1:(end-1))]
%         
%         %Calculate output
%         rateRPM = abs((frame*weight_Vector)./(12*ts));
%         if (rateRPM > 400000)
%             rateRPM = single(0);
%         end
%         
%     end
% end


%     
% double sg_filter(const double raw_data[5])
% {
%     const int i = 2;
%     double result(0);
%     
%     result = (1.0/35.0) * ( - 3.0*raw_data[i-2]  
%                             + 12.0*raw_data[i-1]
%                             + 17.0*raw_data[i]  
%                             + 12.0*raw_data[i+1] 
%                             - 3.0*raw_data[i+2] );
%     return result;
% }
%         
%     
%     

        
    
        
        



            
    %ONE WHEEL AT FRONT AND ONE AT REAR IS INACCURATE.
    % If Fz left > Fz right AND left_Var < limit  -> trust left wheels
    % If Fz right < Fz right AND right_Var < limit -> trust right wheels
    
    %TWO WHEELS AT EITHER FRONT OR REAR ARE WRONG
    
    
    %
        
    % Find Gains in K
    % Hvis alle er ca samme, høy gain
    % Hvis front/rear left/right er forskjellige, stol på de to med mest
    % normalkrefter 
    
    % Essensen er: Hvis fysiske conditions tilsier at hjulfart = bilfart,
    % sett høy Ki. 
    
    % Variansen av et sett med målinger for ett hjul ? 
    
    % Ta covariansen for ax run?
    % Covariance for skidpad run?
    
    
    % If all wheels are approx the same, I still need to check for 
    % physical stuff, such as how fast the rpm is increasing.
    
    %Acceleration:
    %All wheels can slip hence max rate of change is valid 
   
    %Skidpad:
    %All wheels can slip at start
    %If negative torque, braking slip can occur.. 
    
    
    % If front / rear are pretty equal, then since variance of all is
    % pretty high. Must imply that either F_LR or R_LR, or (F_LR && R_LR)
    % is high.
    
    % One wheel is spinning ( FL) , total var is high, FR var > limit
    % -> low var rear , high var front. trust only rear wheels.
